simulink model "Robot9"  (R2025b)
settings: Solver=VariableStepAuto  StartTime=0.0  StopTime=5800  FixedStep=0.01  RelTol=1e-3
undefined symbols (not defined in the file): Brick_x, Brick_y, Brick_z, C_tile_force, C_tile_torque, Container_x, Container_y, Container_z, J_B_B_SIM, J_C_C_SIM, J_P_P_SIM, J_T_T_SIM, K_aocs_tuned, K_arm_tuned, K_tile_force, K_tile_torque, m_B_SIM, m_C_SIM, m_P_SIM, m_T_SIM, robot, X, Y, Z
libraries: nesl_utility x201, sm_lib x116, My_Kinematics_Library x2, simulink_extras x2, dspmathops x1
(part 8 of 8)

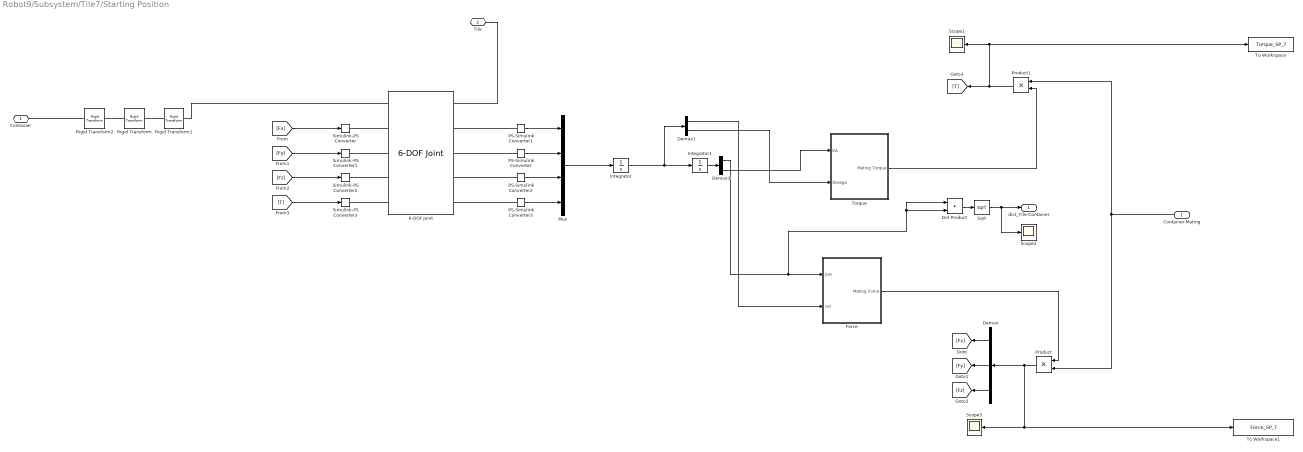
== system Robot9/Subsystem/Tile7/Starting Position ==
  Container Mating : Inport
  6-DOF Joint : sm_lib/Joints/6-DOF Joint  JointMode=Normal  CompositeWrenchDir=FollowerOnBase  CompositeWrenchFrame=BaseFrame  SenseConstraintForce=off  SenseConstraintTorque=off  SenseTotalForce=off  SenseTotalTorque=off  PxPositionTargetSpecify=off  PxPositionTargetPriority=High  PxPositionTargetValue=0  PxPositionTargetValueUnits=m  PxVelocityTargetSpecify=off  PxVelocityTargetPriority=High  PxVelocityTargetValue=0  PxVelocityTargetValueUnits=m/s  PxEquilibriumPosition=0  PxEquilibriumPositionUnits=m  PxSpringStiffness=0  PxSpringStiffnessUnits=N/m  PxDampingCoefficient=0  PxDampingCoefficientUnits=N/(m/s)  PxLowerLimitSpecify=off  PxLowerLimitBound=-1  PxLowerLimitBoundUnits=m  PxLowerLimitStiffness=1e6  PxLowerLimitStiffnessUnits=N/m  PxLowerLimitDamping=1e3  PxLowerLimitDampingUnits=N/(m/s)  PxLowerLimitTransitionRegionWidth=1e-4  PxLowerLimitTransitionRegionWidthUnits=m  PxUpperLimitSpecify=off  PxUpperLimitBound=1  PxUpperLimitBoundUnits=m  PxUpperLimitStiffness=1e6  PxUpperLimitStiffnessUnits=N/m  PxUpperLimitDamping=1e3  PxUpperLimitDampingUnits=N/(m/s)  PxUpperLimitTransitionRegionWidth=1e-4  PxUpperLimitTransitionRegionWidthUnits=m  PxTorqueActuationMode=InputTorque  PxMotionActuationMode=ComputedMotion  PxSensePosition=off  PxSenseVelocity=off  PxSenseAcceleration=on  PxSenseTorqueForce=off  PxSenseLowerLimitTorqueForce=off  PxSenseUpperLimitTorqueForce=off  PyPositionTargetSpecify=off  PyPositionTargetPriority=High  PyPositionTargetValue=0  PyPositionTargetValueUnits=m  PyVelocityTargetSpecify=off  PyVelocityTargetPriority=High  PyVelocityTargetValue=0  PyVelocityTargetValueUnits=m/s  PyEquilibriumPosition=0  PyEquilibriumPositionUnits=m  PySpringStiffness=0  PySpringStiffnessUnits=N/m  PyDampingCoefficient=0  PyDampingCoefficientUnits=N/(m/s)  PyLowerLimitSpecify=off  PyLowerLimitBound=-1  PyLowerLimitBoundUnits=m  PyLowerLimitStiffness=1e6  PyLowerLimitStiffnessUnits=N/m  PyLowerLimitDamping=1e3  PyLowerLimitDampingUnits=N/(m/s)  PyLowerLimitTransitionRegionWidth=1e-4  PyLowerLimitTransitionRegionWidthUnits=m  PyUpperLimitSpecify=off  PyUpperLimitBound=1  PyUpperLimitBoundUnits=m  PyUpperLimitStiffness=1e6  PyUpperLimitStiffnessUnits=N/m  PyUpperLimitDamping=1e3  PyUpperLimitDampingUnits=N/(m/s)  PyUpperLimitTransitionRegionWidth=1e-4  PyUpperLimitTransitionRegionWidthUnits=m  PyTorqueActuationMode=InputTorque  PyMotionActuationMode=ComputedMotion  PySensePosition=off  PySenseVelocity=off  PySenseAcceleration=on  PySenseTorqueForce=off  PySenseLowerLimitTorqueForce=off  PySenseUpperLimitTorqueForce=off  PzPositionTargetSpecify=off  PzPositionTargetPriority=High  PzPositionTargetValue=0  PzPositionTargetValueUnits=m  PzVelocityTargetSpecify=off  PzVelocityTargetPriority=High  PzVelocityTargetValue=0  PzVelocityTargetValueUnits=m/s  PzEquilibriumPosition=0  PzEquilibriumPositionUnits=m  PzSpringStiffness=0  PzSpringStiffnessUnits=N/m  PzDampingCoefficient=0  PzDampingCoefficientUnits=N/(m/s)  PzLowerLimitSpecify=off  PzLowerLimitBound=-1  PzLowerLimitBoundUnits=m  PzLowerLimitStiffness=1e6  PzLowerLimitStiffnessUnits=N/m  PzLowerLimitDamping=1e3  PzLowerLimitDampingUnits=N/(m/s)  PzLowerLimitTransitionRegionWidth=1e-4  PzLowerLimitTransitionRegionWidthUnits=m  PzUpperLimitSpecify=off  PzUpperLimitBound=1  PzUpperLimitBoundUnits=m  PzUpperLimitStiffness=1e6  PzUpperLimitStiffnessUnits=N/m  PzUpperLimitDamping=1e3  PzUpperLimitDampingUnits=N/(m/s)  PzUpperLimitTransitionRegionWidth=1e-4  PzUpperLimitTransitionRegionWidthUnits=m  PzTorqueActuationMode=InputTorque  PzMotionActuationMode=ComputedMotion  PzSensePosition=off  PzSenseVelocity=off  PzSenseAcceleration=on  PzSenseTorqueForce=off  PzSenseLowerLimitTorqueForce=off  PzSenseUpperLimitTorqueForce=off  SphPositionTargetSpecify=off  SphPositionTargetPriority=High  SphPositionTargetRotationMethod=None  SphPositionTargetFollAlignAxisA=+X  SphPositionTargetBaseAlignAxisA=+Y  SphPositionTargetFollAlignAxisB=+Y  SphPositionTargetBaseAlignAxisB=+Z  SphPositionTargetRotationStandardAxis=+Z  SphPositionTargetRotationAngle=0  SphPositionTargetRotationAngleUnits=deg  SphPositionTargetRotationArbitraryAxis=[0 0 1]  SphPositionTargetRotationSequenceAxes=FollowerAxes  SphPositionTargetRotationSequence=XYX  SphPositionTargetRotationSequenceAngles=[0 0 0]  SphPositionTargetRotationSequenceAnglesUnits=deg  SphPositionTargetRotationMatrix=[1 0 0;0 1 0;0 0 1]  SphPositionTargetQuaternion=[1 0 0 0]  SphVelocityTargetSpecify=off  SphVelocityTargetPriority=High  SphVelocityTargetValue=[0 0 0]  SphVelocityTargetValueUnits=deg/s  SphVelocityTargetInFollowerFrame=on  SphEqPosRotationMethod=None  SphEqPosFollAlignAxisA=+X  SphEqPosBaseAlignAxisA=+Y  SphEqPosFollAlignAxisB=+Y  SphEqPosBaseAlignAxisB=+Z  SphEqPosRotationStandardAxis=+Z  SphEqPosRotationAngle=0  SphEqPosRotationAngleUnits=deg  SphEqPosRotationArbitraryAxis=[0 0 1]  SphEqPosRotationSequenceAxes=FollowerAxes  SphEqPosRotationSequence=XYX  SphEqPosRotationSequenceAngles=[0 0 0]  SphEqPosRotationSequenceAnglesUnits=deg  SphEqPosRotationMatrix=[1 0 0;0 1 0;0 0 1]  SphEqPosQuaternion=[1 0 0 0]  SphSpringStiffness=0  SphSpringStiffnessUnits=N*m/deg  SphDampingCoefficient=0  SphDampingCoefficientUnits=N*m/(deg/s)  SphLowerLimitSpecify=off  SphLowerLimitBound=15  SphLowerLimitBoundUnits=deg  SphLowerLimitStiffness=1e4  SphLowerLimitStiffnessUnits=N*m/deg  SphLowerLimitDamping=10  SphLowerLimitDampingUnits=N*m/(deg/s)  SphLowerLimitTransitionRegionWidth=0.1  SphLowerLimitTransitionRegionWidthUnits=deg  SphUpperLimitSpecify=off  SphUpperLimitBound=45  SphUpperLimitBoundUnits=deg  SphUpperLimitStiffness=1e4  SphUpperLimitStiffnessUnits=N*m/deg  SphUpperLimitDamping=10  SphUpperLimitDampingUnits=N*m/(deg/s)  SphUpperLimitTransitionRegionWidth=0.1  SphUpperLimitTransitionRegionWidthUnits=deg  SphTorqueActuationMode=InputTorque  SphActuateTorqueX=off  SphActuateTorqueY=off  SphActuateTorqueZ=off  SphActuateTorque=on  SphActuationFrame=BaseFrame  SphSensePosition=off  SphSenseVelocityX=off  SphSenseVelocityY=off  SphSenseVelocityZ=off  SphSenseVelocity=off  SphSenseAccelerationX=off  SphSenseAccelerationY=off  SphSenseAccelerationZ=off  SphSenseAcceleration=on  SphSenseLowerLimitTorqueMag=off  SphSenseUpperLimitTorqueMag=off  SphSensingFrame=BaseFrame
  Demux : Demux  Outputs=3
  Demux1 : Demux  Outputs=2
  Demux3 : Demux  Outputs=2
  Dot Product : DotProduct  OutDataTypeStr=Inherit: Inherit via internal rule
  Force : Subsystem
  Integrator : Integrator
  Integrator1 : Integrator
  Mux : Mux
  PS-Simulink Converter{,1..3} (4 alike) : nesl_utility/PS-Simulink Converter  PhysicalDomain=network_engine_domain  SubClassName=ps_output  LeftPortType=input  RightPortType=output  PseudoPeriodic=off  Frequencies=[]  VectorFormat=inherit  Unit=inherit  AffineConversion=off
  Product : Product
  Product1 : Product
  Rigid Transform : sm_lib/Frames and Transforms/Rigid Transform  RotationMethod=RotationMatrix  FollAlignAxisA=+X  BaseAlignAxisA=+Y  FollAlignAxisB=+Y  BaseAlignAxisB=+Z  RotationStandardAxis=+Z  RotationAngle=0  RotationAngleUnits=deg  RotationArbitraryAxis=[0 0 1]  RotationSequenceAxes=FollowerAxes  RotationSequence=XYX  RotationSequenceAngles=[0 0 0]  RotationSequenceAnglesUnits=deg  RotationMatrix=[0 0 1;0 1 0;-1 0 0]  Quaternion=[1 0 0 0]  TranslationMethod=None  TranslationCartesianOffset=[0 0 0]  TranslationCartesianOffsetUnits=m  TranslationStandardAxis=+Z  TranslationStandardOffset=0  TranslationStandardOffsetUnits=m  TranslationROffset=0  TranslationROffsetUnits=m  TranslationThetaOffset=0  TranslationThetaOffsetUnits=deg  TranslationZOffset=0  TranslationZOffsetUnits=m
  Rigid Transform1 : sm_lib/Frames and Transforms/Rigid Transform  RotationMethod=StandardAxis  FollAlignAxisA=+X  BaseAlignAxisA=+Y  FollAlignAxisB=+Y  BaseAlignAxisB=+Z  RotationStandardAxis=+Z  RotationAngle=90  RotationAngleUnits=deg  RotationArbitraryAxis=[0 0 1]  RotationSequenceAxes=FollowerAxes  RotationSequence=XYX  RotationSequenceAngles=[0 0 0]  RotationSequenceAnglesUnits=deg  RotationMatrix=[0 0 1;0 1 0;-1 0 0]  Quaternion=[1 0 0 0]  TranslationMethod=None  TranslationCartesianOffset=[0 0 0]  TranslationCartesianOffsetUnits=m  TranslationStandardAxis=+Z  TranslationStandardOffset=0  TranslationStandardOffsetUnits=m  TranslationROffset=0  TranslationROffsetUnits=m  TranslationThetaOffset=0  TranslationThetaOffsetUnits=deg  TranslationZOffset=0  TranslationZOffsetUnits=m
  Rigid Transform2 : sm_lib/Frames and Transforms/Rigid Transform  RotationMethod=None  FollAlignAxisA=+X  BaseAlignAxisA=+Y  FollAlignAxisB=+Y  BaseAlignAxisB=+Z  RotationStandardAxis=+Z  RotationAngle=0  RotationAngleUnits=deg  RotationArbitraryAxis=[0 0 1]  RotationSequenceAxes=FollowerAxes  RotationSequence=XYX  RotationSequenceAngles=[0 0 0]  RotationSequenceAnglesUnits=deg  RotationMatrix=[0 0 1;0 1 0;-1 0 0]  Quaternion=[1 0 0 0]  TranslationMethod=StandardAxis  TranslationCartesianOffset=[0 0 0]  TranslationCartesianOffsetUnits=m  TranslationStandardAxis=-X  TranslationStandardOffset=1.4  TranslationStandardOffsetUnits=m  TranslationROffset=0  TranslationROffsetUnits=m  TranslationThetaOffset=0  TranslationThetaOffsetUnits=deg  TranslationZOffset=0  TranslationZOffsetUnits=m
  Scope1 : Scope
      settings: ActiveDisplayYMinimum=-0.37609374361121245  ActiveDisplayYMaximum=0.37067192520647524  DataLoggingVariableName=ScopeData2
  Scope2 : Scope
      settings: ActiveDisplayYMinimum=-1.5726948982694345E-7  ActiveDisplayYMaximum=1.4154254084424912E-6  DataLoggingVariableName=ScopeData3
  Scope3 : Scope
      settings: ActiveDisplayYMinimum=-3.5066921749591584  ActiveDisplayYMaximum=2.5219185442948877  DataLoggingVariableName=ScopeData4
  Simulink-PS Converter{,1..3} (4 alike) : nesl_utility/Simulink-PS Converter  PhysicalDomain=network_engine_domain  SubClassName=ps_input  LeftPortType=input  RightPortType=output  PseudoPeriodic=off  Frequencies=[]  NoiseDistribution=none  NoiseParameters=[]  Unit=1  AffineConversion=off  FilteringAndDerivatives=provide  SimscapeFilterOrder=1  InputFilterTimeConstant=0.001  UdotUserProvided=0
  Sqrt : Sqrt
  To Workspace : ToWorkspace  VariableName=Torque_SP_7  SaveFormat=Timeseries  SampleTime=-1
  To Workspace1 : ToWorkspace  VariableName=Force_SP_7  SaveFormat=Timeseries  SampleTime=-1
  Torque : Subsystem
  Container : PMIOPort  Side=Left
  Tile : PMIOPort  Port=2  Side=Left
  dist_Tile-Container : Outport
  wires:
  Demux/2 -> [Fy]
  Force/1(Mating Force) -> Product/1
  Demux/1 -> [Fx]
  Demux/3 -> [Fz]
  Container Mating/1 -> Product/2, Product1/1
  Dot Product/1 -> Sqrt/1
  Sqrt/1 -> Scope2/1, dist_Tile-Container/1
  Torque/1(Mating Torque) -> Product1/2
  Integrator1/1 -> Demux3/1
  Demux1/2 -> Torque/2(Omega)
  Demux3/2 -> Torque/1(EA)
  Demux1/1 -> Force/2(vel)
  [Fy] -> Simulink-PS Converter1/1
  [Fx] -> Simulink-PS Converter/1
  Demux3/1 -> Dot Product/2, Dot Product/1, Force/1(pos)
  PS-Simulink Converter2/1 -> Mux/3
  PS-Simulink Converter3/1 -> Mux/4
  [T] -> Simulink-PS Converter3/1
  [Fz] -> Simulink-PS Converter2/1
  PS-Simulink Converter1/1 -> Mux/1
  Integrator/1 -> Demux1/1, Integrator1/1
  Mux/1 -> Integrator/1
  PS-Simulink Converter/1 -> Mux/2
  Product1/1 -> To Workspace/1, Scope1/1, [T]
  Product/1 -> To Workspace1/1, Scope3/1, Demux/1
  connections:
  PS-Simulink Converter3/LConn1 -- 6-DOF Joint/RConn5
  6-DOF Joint/LConn4 -- Simulink-PS Converter2/RConn1
  PS-Simulink Converter/LConn1 -- 6-DOF Joint/RConn3
  6-DOF Joint/LConn3 -- Simulink-PS Converter1/RConn1
  6-DOF Joint/LConn5 -- Simulink-PS Converter3/RConn1
  6-DOF Joint/LConn1 -- Rigid Transform1/RConn1
  PS-Simulink Converter1/LConn1 -- 6-DOF Joint/RConn2
  Rigid Transform2/LConn1 -- Container/RConn1
  6-DOF Joint/LConn2 -- Simulink-PS Converter/RConn1
  Tile/RConn1 -- 6-DOF Joint/RConn1
  Rigid Transform1/LConn1 -- Rigid Transform/RConn1
  Rigid Transform/LConn1 -- Rigid Transform2/RConn1
  PS-Simulink Converter2/LConn1 -- 6-DOF Joint/RConn4

== system Robot9/Subsystem/Tile1/Depose/Force ==
  pos : Inport
  vel : Inport  Port=2
  Constant : Constant  Value=K_tile_force
  Constant1 : Constant  Value=C_tile_force
  Product : Product
  Product1 : Product
  Sum : Sum  Inputs=--
  Mating : Outport
  wires:
  vel/1 -> Product1/1
  pos/1 -> Product/2
  Sum/1 -> Mating/1
  Product1/1 -> Sum/2
  Product/1 -> Sum/1
  Constant1/1 -> Product1/2
  Constant/1 -> Product/1

== system Robot9/Subsystem/Tile1/Depose/Torque ==
  EA : Inport
  Omega : Inport  Port=2
  Constant : Constant  Value=K_tile_torque
  Constant1 : Constant  Value=C_tile_torque
  Product : Product
  Product1 : Product
  Sum : Sum  Inputs=--
  Mating : Outport
  wires:
  Constant/1 -> Product/1
  Constant1/1 -> Product1/2
  Product/1 -> Sum/1
  Product1/1 -> Sum/2
  Sum/1 -> Mating/1
  EA/1 -> Product/2
  Omega/1 -> Product1/1

== system Robot9/Subsystem/Tile1/Grab/Force ==
  pos : Inport
  vel : Inport  Port=2
  Constant : Constant  Value=K_tile_force
  Constant1 : Constant  Value=C_tile_force
  Product : Product
  Product1 : Product
  Sum : Sum  Inputs=--
  Mating : Outport
  wires:
  Constant/1 -> Product/1
  Constant1/1 -> Product1/2
  Product/1 -> Sum/1
  Product1/1 -> Sum/2
  Sum/1 -> Mating/1
  pos/1 -> Product/2
  vel/1 -> Product1/1

== system Robot9/Subsystem/Tile1/Grab/Torque ==
  EA : Inport
  Omega : Inport  Port=2
  Constant : Constant  Value=K_tile_torque
  Constant1 : Constant  Value=C_tile_torque
  Product : Product
  Product1 : Product
  Sum : Sum  Inputs=--
  Mating : Outport
  wires:
  Omega/1 -> Product1/1
  EA/1 -> Product/2
  Sum/1 -> Mating/1
  Product1/1 -> Sum/2
  Product/1 -> Sum/1
  Constant1/1 -> Product1/2
  Constant/1 -> Product/1

== system Robot9/Subsystem/Tile1/Starting Position/Force ==
  pos : Inport
  vel : Inport  Port=2
  Constant : Constant  Value=K_tile_force
  Constant1 : Constant  Value=C_tile_force
  Product : Product
  Product1 : Product
  Sum : Sum  Inputs=--
  Mating Force : Outport
  wires:
  Constant/1 -> Product/1
  Constant1/1 -> Product1/2
  Product/1 -> Sum/1
  Product1/1 -> Sum/2
  Sum/1 -> Mating Force/1
  pos/1 -> Product/2
  vel/1 -> Product1/1

== system Robot9/Subsystem/Tile1/Starting Position/Torque ==
  EA : Inport
  Omega : Inport  Port=2
  Constant : Constant  Value=K_tile_torque
  Constant1 : Constant  Value=C_tile_torque
  Product : Product
  Product1 : Product
  Sum : Sum  Inputs=--
  Mating Torque : Outport
  wires:
  Omega/1 -> Product1/1
  EA/1 -> Product/2
  Sum/1 -> Mating Torque/1
  Product1/1 -> Sum/2
  Product/1 -> Sum/1
  Constant1/1 -> Product1/2
  Constant/1 -> Product/1

== system Robot9/Subsystem/Tile2/Depose/Force ==
  pos : Inport
  vel : Inport  Port=2
  Constant : Constant  Value=K_tile_force
  Constant1 : Constant  Value=C_tile_force
  Product : Product
  Product1 : Product
  Sum : Sum  Inputs=--
  Mating : Outport
  wires:
  Constant/1 -> Product/1
  Constant1/1 -> Product1/2
  Product/1 -> Sum/1
  Product1/1 -> Sum/2
  Sum/1 -> Mating/1
  pos/1 -> Product/2
  vel/1 -> Product1/1

== system Robot9/Subsystem/Tile2/Depose/Torque ==
  EA : Inport
  Omega : Inport  Port=2
  Constant : Constant  Value=K_tile_torque
  Constant1 : Constant  Value=C_tile_torque
  Product : Product
  Product1 : Product
  Sum : Sum  Inputs=--
  Mating : Outport
  wires:
  Omega/1 -> Product1/1
  EA/1 -> Product/2
  Sum/1 -> Mating/1
  Product1/1 -> Sum/2
  Product/1 -> Sum/1
  Constant1/1 -> Product1/2
  Constant/1 -> Product/1

== system Robot9/Subsystem/Tile2/Grab/Force ==
  pos : Inport
  vel : Inport  Port=2
  Constant : Constant  Value=K_tile_force
  Constant1 : Constant  Value=C_tile_force
  Product : Product
  Product1 : Product
  Sum : Sum  Inputs=--
  Mating : Outport
  wires:
  vel/1 -> Product1/1
  pos/1 -> Product/2
  Sum/1 -> Mating/1
  Product1/1 -> Sum/2
  Product/1 -> Sum/1
  Constant1/1 -> Product1/2
  Constant/1 -> Product/1

== system Robot9/Subsystem/Tile2/Grab/Torque ==
  EA : Inport
  Omega : Inport  Port=2
  Constant : Constant  Value=K_tile_torque
  Constant1 : Constant  Value=C_tile_torque
  Product : Product
  Product1 : Product
  Sum : Sum  Inputs=--
  Mating : Outport
  wires:
  Constant/1 -> Product/1
  Constant1/1 -> Product1/2
  Product/1 -> Sum/1
  Product1/1 -> Sum/2
  Sum/1 -> Mating/1
  EA/1 -> Product/2
  Omega/1 -> Product1/1

== system Robot9/Subsystem/Tile2/Starting Position/Force ==
  pos : Inport
  vel : Inport  Port=2
  Constant : Constant  Value=K_tile_force
  Constant1 : Constant  Value=C_tile_force
  Product : Product
  Product1 : Product
  Sum : Sum  Inputs=--
  Mating Force : Outport
  wires:
  Constant/1 -> Product/1
  Constant1/1 -> Product1/2
  Product/1 -> Sum/1
  Product1/1 -> Sum/2
  Sum/1 -> Mating Force/1
  pos/1 -> Product/2
  vel/1 -> Product1/1

== system Robot9/Subsystem/Tile2/Starting Position/Torque ==
  EA : Inport
  Omega : Inport  Port=2
  Constant : Constant  Value=K_tile_torque
  Constant1 : Constant  Value=C_tile_torque
  Product : Product
  Product1 : Product
  Sum : Sum  Inputs=--
  Mating Torque : Outport
  wires:
  Omega/1 -> Product1/1
  EA/1 -> Product/2
  Sum/1 -> Mating Torque/1
  Product1/1 -> Sum/2
  Product/1 -> Sum/1
  Constant1/1 -> Product1/2
  Constant/1 -> Product/1

== system Robot9/Subsystem/Tile3/Depose/Force ==
  pos : Inport
  vel : Inport  Port=2
  Constant : Constant  Value=K_tile_force
  Constant1 : Constant  Value=C_tile_force
  Product : Product
  Product1 : Product
  Sum : Sum  Inputs=--
  Mating : Outport
  wires:
  vel/1 -> Product1/1
  pos/1 -> Product/2
  Sum/1 -> Mating/1
  Product1/1 -> Sum/2
  Product/1 -> Sum/1
  Constant1/1 -> Product1/2
  Constant/1 -> Product/1

== system Robot9/Subsystem/Tile3/Depose/Torque ==
  EA : Inport
  Omega : Inport  Port=2
  Constant : Constant  Value=K_tile_torque
  Constant1 : Constant  Value=C_tile_torque
  Product : Product
  Product1 : Product
  Sum : Sum  Inputs=--
  Mating : Outport
  wires:
  Constant/1 -> Product/1
  Constant1/1 -> Product1/2
  Product/1 -> Sum/1
  Product1/1 -> Sum/2
  Sum/1 -> Mating/1
  EA/1 -> Product/2
  Omega/1 -> Product1/1

== system Robot9/Subsystem/Tile3/Grab/Force ==
  pos : Inport
  vel : Inport  Port=2
  Constant : Constant  Value=K_tile_force
  Constant1 : Constant  Value=C_tile_force
  Product : Product
  Product1 : Product
  Sum : Sum  Inputs=--
  Mating : Outport
  wires:
  Constant/1 -> Product/1
  Constant1/1 -> Product1/2
  Product/1 -> Sum/1
  Product1/1 -> Sum/2
  Sum/1 -> Mating/1
  pos/1 -> Product/2
  vel/1 -> Product1/1

== system Robot9/Subsystem/Tile3/Grab/Torque ==
  EA : Inport
  Omega : Inport  Port=2
  Constant : Constant  Value=K_tile_torque
  Constant1 : Constant  Value=C_tile_torque
  Product : Product
  Product1 : Product
  Sum : Sum  Inputs=--
  Mating : Outport
  wires:
  Omega/1 -> Product1/1
  EA/1 -> Product/2
  Sum/1 -> Mating/1
  Product1/1 -> Sum/2
  Product/1 -> Sum/1
  Constant1/1 -> Product1/2
  Constant/1 -> Product/1

== system Robot9/Subsystem/Tile3/Starting Position/Force ==
  pos : Inport
  vel : Inport  Port=2
  Constant : Constant  Value=150000
  Constant1 : Constant  Value=8000
  Product : Product
  Product1 : Product
  Sum : Sum  Inputs=--
  Mating Force : Outport
  wires:
  Constant/1 -> Product/1
  Constant1/1 -> Product1/2
  Product/1 -> Sum/1
  Product1/1 -> Sum/2
  Sum/1 -> Mating Force/1
  pos/1 -> Product/2
  vel/1 -> Product1/1

== system Robot9/Subsystem/Tile3/Starting Position/Torque ==
  EA : Inport
  Omega : Inport  Port=2
  Constant : Constant  Value=150000
  Constant1 : Constant  Value=8000
  Product : Product
  Product1 : Product
  Sum : Sum  Inputs=--
  Mating Torque : Outport
  wires:
  Omega/1 -> Product1/1
  EA/1 -> Product/2
  Sum/1 -> Mating Torque/1
  Product1/1 -> Sum/2
  Product/1 -> Sum/1
  Constant1/1 -> Product1/2
  Constant/1 -> Product/1

== system Robot9/Subsystem/Tile4/Depose/Force ==
  pos : Inport
  vel : Inport  Port=2
  Constant : Constant  Value=K_tile_force
  Constant1 : Constant  Value=C_tile_force
  Product : Product
  Product1 : Product
  Sum : Sum  Inputs=--
  Mating : Outport
  wires:
  Constant/1 -> Product/1
  Constant1/1 -> Product1/2
  Product/1 -> Sum/1
  Product1/1 -> Sum/2
  Sum/1 -> Mating/1
  pos/1 -> Product/2
  vel/1 -> Product1/1

== system Robot9/Subsystem/Tile4/Depose/Torque ==
  EA : Inport
  Omega : Inport  Port=2
  Constant : Constant  Value=K_tile_torque
  Constant1 : Constant  Value=C_tile_torque
  Product : Product
  Product1 : Product
  Sum : Sum  Inputs=--
  Mating : Outport
  wires:
  Omega/1 -> Product1/1
  EA/1 -> Product/2
  Sum/1 -> Mating/1
  Product1/1 -> Sum/2
  Product/1 -> Sum/1
  Constant1/1 -> Product1/2
  Constant/1 -> Product/1

== system Robot9/Subsystem/Tile4/Grab/Force ==
  pos : Inport
  vel : Inport  Port=2
  Constant : Constant  Value=K_tile_force
  Constant1 : Constant  Value=C_tile_force
  Product : Product
  Product1 : Product
  Sum : Sum  Inputs=--
  Mating : Outport
  wires:
  vel/1 -> Product1/1
  pos/1 -> Product/2
  Sum/1 -> Mating/1
  Product1/1 -> Sum/2
  Product/1 -> Sum/1
  Constant1/1 -> Product1/2
  Constant/1 -> Product/1

== system Robot9/Subsystem/Tile4/Grab/Torque ==
  EA : Inport
  Omega : Inport  Port=2
  Constant : Constant  Value=K_tile_torque
  Constant1 : Constant  Value=C_tile_torque
  Product : Product
  Product1 : Product
  Sum : Sum  Inputs=--
  Mating : Outport
  wires:
  Constant/1 -> Product/1
  Constant1/1 -> Product1/2
  Product/1 -> Sum/1
  Product1/1 -> Sum/2
  Sum/1 -> Mating/1
  EA/1 -> Product/2
  Omega/1 -> Product1/1

== system Robot9/Subsystem/Tile4/Starting Position/Force ==
  pos : Inport
  vel : Inport  Port=2
  Constant : Constant  Value=150000
  Constant1 : Constant  Value=8000
  Product : Product
  Product1 : Product
  Sum : Sum  Inputs=--
  Mating Force : Outport
  wires:
  Constant/1 -> Product/1
  Constant1/1 -> Product1/2
  Product/1 -> Sum/1
  Product1/1 -> Sum/2
  Sum/1 -> Mating Force/1
  pos/1 -> Product/2
  vel/1 -> Product1/1

== system Robot9/Subsystem/Tile4/Starting Position/Torque ==
  EA : Inport
  Omega : Inport  Port=2
  Constant : Constant  Value=150000
  Constant1 : Constant  Value=8000
  Product : Product
  Product1 : Product
  Sum : Sum  Inputs=--
  Mating Torque : Outport
  wires:
  Omega/1 -> Product1/1
  EA/1 -> Product/2
  Sum/1 -> Mating Torque/1
  Product1/1 -> Sum/2
  Product/1 -> Sum/1
  Constant1/1 -> Product1/2
  Constant/1 -> Product/1

== system Robot9/Subsystem/Tile5/Depose/Force ==
  pos : Inport
  vel : Inport  Port=2
  Constant : Constant  Value=K_tile_force
  Constant1 : Constant  Value=C_tile_force
  Product : Product
  Product1 : Product
  Sum : Sum  Inputs=--
  Mating : Outport
  wires:
  vel/1 -> Product1/1
  pos/1 -> Product/2
  Sum/1 -> Mating/1
  Product1/1 -> Sum/2
  Product/1 -> Sum/1
  Constant1/1 -> Product1/2
  Constant/1 -> Product/1

== system Robot9/Subsystem/Tile5/Depose/Torque ==
  EA : Inport
  Omega : Inport  Port=2
  Constant : Constant  Value=K_tile_torque
  Constant1 : Constant  Value=C_tile_torque
  Product : Product
  Product1 : Product
  Sum : Sum  Inputs=--
  Mating : Outport
  wires:
  Constant/1 -> Product/1
  Constant1/1 -> Product1/2
  Product/1 -> Sum/1
  Product1/1 -> Sum/2
  Sum/1 -> Mating/1
  EA/1 -> Product/2
  Omega/1 -> Product1/1

== system Robot9/Subsystem/Tile5/Grab/Force ==
  pos : Inport
  vel : Inport  Port=2
  Constant : Constant  Value=K_tile_force
  Constant1 : Constant  Value=C_tile_force
  Product : Product
  Product1 : Product
  Sum : Sum  Inputs=--
  Mating : Outport
  wires:
  Constant/1 -> Product/1
  Constant1/1 -> Product1/2
  Product/1 -> Sum/1
  Product1/1 -> Sum/2
  Sum/1 -> Mating/1
  pos/1 -> Product/2
  vel/1 -> Product1/1

== system Robot9/Subsystem/Tile5/Grab/Torque ==
  EA : Inport
  Omega : Inport  Port=2
  Constant : Constant  Value=K_tile_torque
  Constant1 : Constant  Value=C_tile_torque
  Product : Product
  Product1 : Product
  Sum : Sum  Inputs=--
  Mating : Outport
  wires:
  Omega/1 -> Product1/1
  EA/1 -> Product/2
  Sum/1 -> Mating/1
  Product1/1 -> Sum/2
  Product/1 -> Sum/1
  Constant1/1 -> Product1/2
  Constant/1 -> Product/1

== system Robot9/Subsystem/Tile5/Starting Position/Force ==
  pos : Inport
  vel : Inport  Port=2
  Constant : Constant  Value=150000
  Constant1 : Constant  Value=8000
  Product : Product
  Product1 : Product
  Sum : Sum  Inputs=--
  Mating Force : Outport
  wires:
  Constant/1 -> Product/1
  Constant1/1 -> Product1/2
  Product/1 -> Sum/1
  Product1/1 -> Sum/2
  Sum/1 -> Mating Force/1
  pos/1 -> Product/2
  vel/1 -> Product1/1

== system Robot9/Subsystem/Tile5/Starting Position/Torque ==
  EA : Inport
  Omega : Inport  Port=2
  Constant : Constant  Value=150000
  Constant1 : Constant  Value=8000
  Product : Product
  Product1 : Product
  Sum : Sum  Inputs=--
  Mating Torque : Outport
  wires:
  Omega/1 -> Product1/1
  EA/1 -> Product/2
  Sum/1 -> Mating Torque/1
  Product1/1 -> Sum/2
  Product/1 -> Sum/1
  Constant1/1 -> Product1/2
  Constant/1 -> Product/1

== system Robot9/Subsystem/Tile6/Depose/Force ==
  pos : Inport
  vel : Inport  Port=2
  Constant : Constant  Value=K_tile_force
  Constant1 : Constant  Value=C_tile_force
  Product : Product
  Product1 : Product
  Sum : Sum  Inputs=--
  Mating : Outport
  wires:
  Constant/1 -> Product/1
  Constant1/1 -> Product1/2
  Product/1 -> Sum/1
  Product1/1 -> Sum/2
  Sum/1 -> Mating/1
  pos/1 -> Product/2
  vel/1 -> Product1/1

== system Robot9/Subsystem/Tile6/Depose/Torque ==
  EA : Inport
  Omega : Inport  Port=2
  Constant : Constant  Value=K_tile_torque
  Constant1 : Constant  Value=C_tile_torque
  Product : Product
  Product1 : Product
  Sum : Sum  Inputs=--
  Mating : Outport
  wires:
  Omega/1 -> Product1/1
  EA/1 -> Product/2
  Sum/1 -> Mating/1
  Product1/1 -> Sum/2
  Product/1 -> Sum/1
  Constant1/1 -> Product1/2
  Constant/1 -> Product/1

== system Robot9/Subsystem/Tile6/Grab/Force ==
  pos : Inport
  vel : Inport  Port=2
  Constant : Constant  Value=K_tile_force
  Constant1 : Constant  Value=C_tile_force
  Product : Product
  Product1 : Product
  Sum : Sum  Inputs=--
  Mating : Outport
  wires:
  vel/1 -> Product1/1
  pos/1 -> Product/2
  Sum/1 -> Mating/1
  Product1/1 -> Sum/2
  Product/1 -> Sum/1
  Constant1/1 -> Product1/2
  Constant/1 -> Product/1

== system Robot9/Subsystem/Tile6/Grab/Torque ==
  EA : Inport
  Omega : Inport  Port=2
  Constant : Constant  Value=K_tile_torque
  Constant1 : Constant  Value=C_tile_torque
  Product : Product
  Product1 : Product
  Sum : Sum  Inputs=--
  Mating : Outport
  wires:
  Constant/1 -> Product/1
  Constant1/1 -> Product1/2
  Product/1 -> Sum/1
  Product1/1 -> Sum/2
  Sum/1 -> Mating/1
  EA/1 -> Product/2
  Omega/1 -> Product1/1

== system Robot9/Subsystem/Tile6/Starting Position/Force ==
  pos : Inport
  vel : Inport  Port=2
  Constant : Constant  Value=150000
  Constant1 : Constant  Value=8000
  Product : Product
  Product1 : Product
  Sum : Sum  Inputs=--
  Mating Force : Outport
  wires:
  Constant/1 -> Product/1
  Constant1/1 -> Product1/2
  Product/1 -> Sum/1
  Product1/1 -> Sum/2
  Sum/1 -> Mating Force/1
  pos/1 -> Product/2
  vel/1 -> Product1/1

== system Robot9/Subsystem/Tile6/Starting Position/Torque ==
  EA : Inport
  Omega : Inport  Port=2
  Constant : Constant  Value=150000
  Constant1 : Constant  Value=8000
  Product : Product
  Product1 : Product
  Sum : Sum  Inputs=--
  Mating Torque : Outport
  wires:
  Omega/1 -> Product1/1
  EA/1 -> Product/2
  Sum/1 -> Mating Torque/1
  Product1/1 -> Sum/2
  Product/1 -> Sum/1
  Constant1/1 -> Product1/2
  Constant/1 -> Product/1

== system Robot9/Subsystem/Tile7/Depose/Force ==
  pos : Inport
  vel : Inport  Port=2
  Constant : Constant  Value=K_tile_force
  Constant1 : Constant  Value=C_tile_force
  Product : Product
  Product1 : Product
  Sum : Sum  Inputs=--
  Mating : Outport
  wires:
  vel/1 -> Product1/1
  pos/1 -> Product/2
  Sum/1 -> Mating/1
  Product1/1 -> Sum/2
  Product/1 -> Sum/1
  Constant1/1 -> Product1/2
  Constant/1 -> Product/1

== system Robot9/Subsystem/Tile7/Depose/Torque ==
  EA : Inport
  Omega : Inport  Port=2
  Constant : Constant  Value=K_tile_torque
  Constant1 : Constant  Value=C_tile_torque
  Product : Product
  Product1 : Product
  Sum : Sum  Inputs=--
  Mating : Outport
  wires:
  Constant/1 -> Product/1
  Constant1/1 -> Product1/2
  Product/1 -> Sum/1
  Product1/1 -> Sum/2
  Sum/1 -> Mating/1
  EA/1 -> Product/2
  Omega/1 -> Product1/1

== system Robot9/Subsystem/Tile7/Grab/Force ==
  pos : Inport
  vel : Inport  Port=2
  Constant : Constant  Value=K_tile_force
  Constant1 : Constant  Value=C_tile_force
  Product : Product
  Product1 : Product
  Sum : Sum  Inputs=--
  Mating : Outport
  wires:
  Constant/1 -> Product/1
  Constant1/1 -> Product1/2
  Product/1 -> Sum/1
  Product1/1 -> Sum/2
  Sum/1 -> Mating/1
  pos/1 -> Product/2
  vel/1 -> Product1/1

== system Robot9/Subsystem/Tile7/Grab/Torque ==
  EA : Inport
  Omega : Inport  Port=2
  Constant : Constant  Value=K_tile_torque
  Constant1 : Constant  Value=C_tile_torque
  Product : Product
  Product1 : Product
  Sum : Sum  Inputs=--
  Mating : Outport
  wires:
  Omega/1 -> Product1/1
  EA/1 -> Product/2
  Sum/1 -> Mating/1
  Product1/1 -> Sum/2
  Product/1 -> Sum/1
  Constant1/1 -> Product1/2
  Constant/1 -> Product/1

== system Robot9/Subsystem/Tile7/Starting Position/Force ==
  pos : Inport
  vel : Inport  Port=2
  Constant : Constant  Value=150000
  Constant1 : Constant  Value=8000
  Product : Product
  Product1 : Product
  Sum : Sum  Inputs=--
  Mating Force : Outport
  wires:
  Constant/1 -> Product/1
  Constant1/1 -> Product1/2
  Product/1 -> Sum/1
  Product1/1 -> Sum/2
  Sum/1 -> Mating Force/1
  pos/1 -> Product/2
  vel/1 -> Product1/1

== system Robot9/Subsystem/Tile7/Starting Position/Torque ==
  EA : Inport
  Omega : Inport  Port=2
  Constant : Constant  Value=150000
  Constant1 : Constant  Value=8000
  Product : Product
  Product1 : Product
  Sum : Sum  Inputs=--
  Mating Torque : Outport
  wires:
  Omega/1 -> Product1/1
  EA/1 -> Product/2
  Sum/1 -> Mating Torque/1
  Product1/1 -> Sum/2
  Product/1 -> Sum/1
  Constant1/1 -> Product1/2
  Constant/1 -> Product/1

== stateflow chart Robot9/Subsystem/Tile4/One Tile Strategy ==
  state Start
    Container_Mating = 1;
    Arm_Mating = 0;
    Antenna_Mating = 0;
  state Grabbing___carring
    Container_Mating = 0;
    Arm_Mating = 1;
    Antenna_Mating = 0;
  state Deposing
    Container_Mating = 0;
    Arm_Mating = 0;
    Antenna_Mating = 1;
  (default) -> Start
  Start -> Grabbing___carring : [dist_arm <= 0.015 && EA_arm<=10*pi/180]
  Grabbing___carring -> Deposing : [dist_endpoint <= 0.015 && EA_endpoint<=10*pi/180]
  data: dist_endpoint input; EA_endpoint input; dist_arm input; Arm_Mating output; Container_Mating output; Antenna_Mating output; EA_arm input

== stateflow chart Robot9/Subsystem/Tile5/One Tile Strategy ==
  state Start
    Container_Mating = 1;
    Arm_Mating = 0;
    Antenna_Mating = 0;
  state Grabbing___carring
    Container_Mating = 0;
    Arm_Mating = 1;
    Antenna_Mating = 0;
  state Deposing
    Container_Mating = 0;
    Arm_Mating = 0;
    Antenna_Mating = 1;
  (default) -> Start
  Start -> Grabbing___carring : [dist_arm <= 0.015 && EA_arm<=10*pi/180]
  Grabbing___carring -> Deposing : [dist_endpoint <= 0.015 && EA_endpoint<=10*pi/180]
  data: dist_endpoint input; EA_endpoint input; dist_arm input; Arm_Mating output; Container_Mating output; Antenna_Mating output; EA_arm input

== stateflow chart Robot9/Subsystem/Tile6/One Tile Strategy ==
  state Start
    Container_Mating = 1;
    Arm_Mating = 0;
    Antenna_Mating = 0;
  state Grabbing___carring
    Container_Mating = 0;
    Arm_Mating = 1;
    Antenna_Mating = 0;
  state Deposing
    Container_Mating = 0;
    Arm_Mating = 0;
    Antenna_Mating = 1;
  (default) -> Start
  Start -> Grabbing___carring : [dist_arm <= 0.015 && EA_arm<=10*pi/180]
  Grabbing___carring -> Deposing : [dist_endpoint <= 0.015 && EA_endpoint<=10*pi/180]
  data: dist_endpoint input; EA_endpoint input; dist_arm input; Arm_Mating output; Container_Mating output; Antenna_Mating output; EA_arm input

== stateflow chart Robot9/Subsystem/Tile7/One Tile Strategy ==
  state Start
    Container_Mating = 1;
    Arm_Mating = 0;
    Antenna_Mating = 0;
  state Grabbing___carring
    Container_Mating = 0;
    Arm_Mating = 1;
    Antenna_Mating = 0;
  state Deposing
    Container_Mating = 0;
    Arm_Mating = 0;
    Antenna_Mating = 1;
  (default) -> Start
  Start -> Grabbing___carring : [dist_arm <= 0.015 && EA_arm<=10*pi/180]
  Grabbing___carring -> Deposing : [dist_endpoint <= 0.015 && EA_endpoint<=10*pi/180]
  data: dist_endpoint input; EA_endpoint input; dist_arm input; Arm_Mating output; Container_Mating output; Antenna_Mating output; EA_arm input

== stateflow chart Robot9/Subsystem/Tile1/One Tile Strategy ==
  state Start
    Container_Mating = 1;
    Arm_Mating = 0;
    Antenna_Mating = 0;
  state Grabbing___carring
    Container_Mating = 0;
    Arm_Mating = 1;
    Antenna_Mating = 0;
  state Deposing
    Container_Mating = 0;
    Arm_Mating = 0;
    Antenna_Mating = 1;
  (default) -> Start
  Start -> Grabbing___carring : [dist_arm <= 0.015 && EA_arm<=10*pi/180]
  Grabbing___carring -> Deposing : [dist_endpoint <= 0.015 && EA_endpoint<=10*pi/180]
  data: dist_endpoint input; EA_endpoint input; dist_arm input; Arm_Mating output; Container_Mating output; Antenna_Mating output; EA_arm input

== stateflow chart Robot9/Subsystem/Tile2/One Tile Strategy ==
  state Start
    Container_Mating = 1;
    Arm_Mating = 0;
    Antenna_Mating = 0;
  state Grabbing___carring
    Container_Mating = 0;
    Arm_Mating = 1;
    Antenna_Mating = 0;
  state Deposing
    Container_Mating = 0;
    Arm_Mating = 0;
    Antenna_Mating = 1;
  (default) -> Start
  Start -> Grabbing___carring : [dist_arm <= 0.015 && EA_arm<=10*pi/180]
  Grabbing___carring -> Deposing : [dist_endpoint <= 0.015 && EA_endpoint<=10*pi/180]
  data: dist_endpoint input; EA_endpoint input; dist_arm input; Arm_Mating output; Container_Mating output; Antenna_Mating output; EA_arm input

== stateflow chart Robot9/Subsystem/Tile3/One Tile Strategy ==
  state Start
    Container_Mating = 1;
    Arm_Mating = 0;
    Antenna_Mating = 0;
  state Grabbing___carring
    Container_Mating = 0;
    Arm_Mating = 1;
    Antenna_Mating = 0;
  state Deposing
    Container_Mating = 0;
    Arm_Mating = 0;
    Antenna_Mating = 1;
  (default) -> Start
  Start -> Grabbing___carring : [dist_arm <= 0.015 && EA_arm<=10*pi/180]
  Grabbing___carring -> Deposing : [dist_endpoint <= 0.015 && EA_endpoint<=10*pi/180]
  data: dist_endpoint input; EA_endpoint input; dist_arm input; Arm_Mating output; Container_Mating output; Antenna_Mating output; EA_arm input
